simulink library "nif"  (Simulink 8.1)
settings: Solver=ode1  StartTime=0.0  StopTime=Inf  FixedStep=0.001  RelTol=1e-3
PostLoadFcn:
  | , if any(exist('dsrtsu_mdlpostloadfcn', 'file') == [2, 3, 6]), try dsrtsu_mdlpostloadfcn('Execute', bdroot); catch fprintf('Error in PostLoadFcn (dsrtsu_mdlpostloadfcn) for model "%s":\n %s\n', bdroot, lasterr); end, end,
undefined symbols (not defined in the file or in its folder): AACC_VehSpdError_kph, KACC_ACCShortSetTimeGap_s, KACC_DistCtrltNoIntrusionAddDecel_mps2, MACC_ACCDistLookUpDecel_mps2, MACC_ACCDistTBLookUpDecel_mps2
libraries: hcu_lib x2
settings Model: DSRTSU_INTERNAL_RTI_VER=450  DSRTSU_INTERNAL_RTI_TYPE=rti1401  Creator=AT015555  LastModifiedBy=AT015555

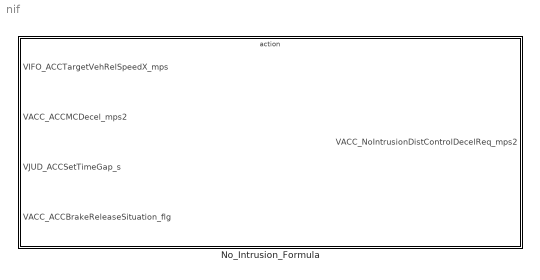
== system nif ==
  No_Intrusion_Formula : Subsystem  TreatAsAtomicUnit=on

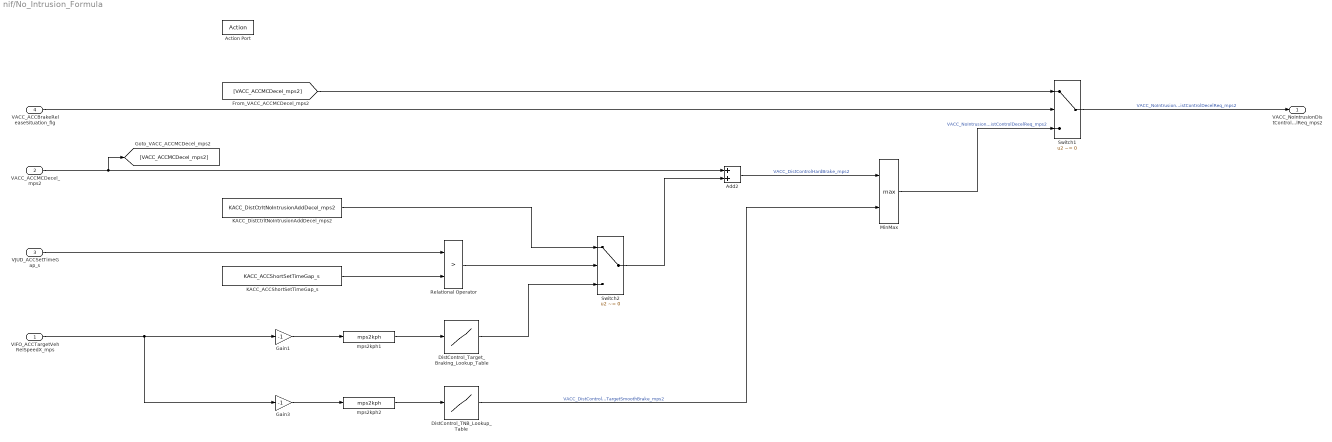
== system nif/No_Intrusion_Formula ==
  VIFO_ACCTargetVehRelSpeedX_mps : Inport
  VACC_ACCMCDecel_mps2 : Inport  Port=2
  VJUD_ACCSetTimeGap_s : Inport  Port=3
  VACC_ACCBrakeReleaseSituation_flg : Inport  Port=4
  Action Port : ActionPort
  Add2 : Sum
  DistControl_TNB_Lookup_Table : Lookup_n-D  NumberOfTableDimensions=1  BreakpointsForDimension1=AACC_VehSpdError_kph  Table=MACC_ACCDistLookUpDecel_mps2  ExtrapMethod=Clip  UseLastTableValue=on  RndMeth=Simplest  InputSameDT=on
  DistControl_Target_Braking_Lookup_Table : Lookup_n-D  NumberOfTableDimensions=1  BreakpointsForDimension1=AACC_VehSpdError_kph  Table=MACC_ACCDistTBLookUpDecel_mps2  ExtrapMethod=Clip  UseLastTableValue=on  RndMeth=Simplest  InputSameDT=on
  Gain1 : Gain  Gain=-1
  Gain3 : Gain  Gain=-1
  KACC_ACCShortSetTimeGap_s : Constant  Value=KACC_ACCShortSetTimeGap_s
  KACC_DistCtrltNoIntrusionAddDecel_mps2 : Constant  Value=KACC_DistCtrltNoIntrusionAddDecel_mps2
  MinMax : MinMax  Function=max  Inputs=2
  Relational Operator : RelationalOperator  Operator=>  OutDataTypeStr=boolean
  Switch1 : Switch  Criteria=u2 ~= 0
  Switch2 : Switch  Criteria=u2 ~= 0
  mps2kph1 : hcu_lib/mps2kph
  mps2kph2 : hcu_lib/mps2kph
  VACC_NoIntrusionDistControlDecelReq_mps2 : Outport
  wires:
  Switch1/1 -> VACC_NoIntrusionDistControlDecelReq_mps2/1  "VACC_NoIntrusionDistControlDecelReq_mps2"
  Gain1/1 -> mps2kph1/1
  mps2kph1/1 -> DistControl_Target_Braking_Lookup_Table/1
  VACC_ACCMCDecel_mps2/1 -> [VACC_ACCMCDecel_mps2], Add2/1
  mps2kph2/1 -> DistControl_TNB_Lookup_Table/1
  Gain3/1 -> mps2kph2/1
  VIFO_ACCTargetVehRelSpeedX_mps/1 -> Gain1/1, Gain3/1
  Add2/1 -> MinMax/1  "VACC_DistControlHardBrake_mps2"
  DistControl_TNB_Lookup_Table/1 -> MinMax/2  "VACC_DistControlTargetSmoothBrake_mps2"
  KACC_DistCtrltNoIntrusionAddDecel_mps2/1 -> Switch2/1
  Relational Operator/1 -> Switch2/2
  VJUD_ACCSetTimeGap_s/1 -> Relational Operator/1
  KACC_ACCShortSetTimeGap_s/1 -> Relational Operator/2
  Switch2/1 -> Add2/2
  DistControl_Target_Braking_Lookup_Table/1 -> Switch2/3
  VACC_ACCBrakeReleaseSituation_flg/1 -> Switch1/2
  MinMax/1 -> Switch1/3  "VACC_NoIntrusionDistControlDecelReq_mps2"
  [VACC_ACCMCDecel_mps2] -> Switch1/1
